simulink model "dspwavelet_frame2"  (R2016b)
settings: Solver=FixedStepDiscrete  StartTime=0.0  StopTime=1024  FixedStep=1e-5  RelTol=1e-3  EnableMultiTasking=on
undefined symbols (not defined in the file or in its folder): lod, ts
libraries: dspsrcs4 x3, dspmlti4 x2, dspmisc x1
settings Model: ExtModeTrigMode=oneshot  ExtModeArmWhenConnect=off  Creator=The MathWorks, Inc.  LastModifiedBy=admin
settings DataIOCC: SaveFormat=Array  SaveOutput=off  SaveTime=off  SignalLoggingName=sigsOut
settings OptimizationCC: BlockReduction=off  BooleanDataType=off  ExpressionDepthLimit=2147483647  InitFltsAndDblsToZero=on  EfficientMapNaN2IntZero=off  LifeSpan=inf
settings DebuggingCC: SaveWithParameterizedLinksMsg=none  UnderspecifiedInitializationDetection=Classic  MergeDetectMultiDrivingBlocksExec=none  SignalResolutionControl=TryResolveAllWithWarning  MultiTaskDSMMsg=warning  MultiTaskCondExecSysMsg=none  IntegerOverflowMsg=none  FcnCallInpInsideContextMsg=warning  StateNameClashWarn=warning  SFUnexpectedBacktrackingDiag=warning  SFNoUnconditionalDefaultTransitionDiag=warning  SFExecutionAtInitializationDiag=none  IntegerSaturationMsg=none
settings HardwareCC: ProdBitPerPointer=32  ProdBitPerSizeT=32  ProdBitPerPtrDiffT=32  ProdLargestAtomicFloat=None  ProdIntDivRoundTo=Undefined  ProdEndianess=Unspecified  ProdWordSize=32  ProdHWDeviceType=32-bit Generic  TargetUnknown=on
settings ModelReferenceCC: PropagateSignalLabelsOutOfModel=off
settings GRTTargetCC: TargetFcnLib=ansi_tfl_tmw.mat  TargetLangStandard=C89/C90 (ANSI)  GeneratePreprocessorConditionals=Disable all  CombineOutputUpdateFcns=off  GRTInterface=on
settings ConfigComp: CovMetricSettings=dw  CovHtmlReporting=on  CovSaveCumulativeToWorkspaceVar=on  CovSaveSingleToWorkspaceVar=on  CovExternalEMLEnable=off  CovSFcnEnable=off

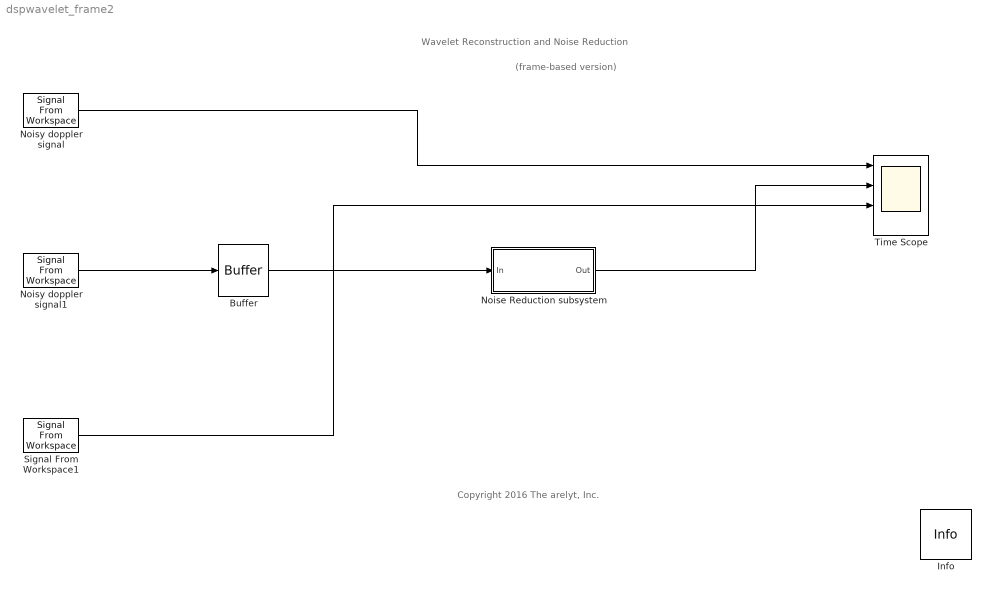
== system dspwavelet_frame2 ==
  note: Wavelet Reconstruction and Noise Reduction
  note: Copyright 2016 The arelyt, Inc.
  note: (frame-based version)
  Buffer : Buffer  TreatMby1Signals=One channel  OutputFrames=off
  Info : dspmisc/Info  SystemSampleTime=-1
  Noise Reduction subsystem : Subsystem  TreatAsAtomicUnit=on
  Noisy doppler signal : dspsrcs4/Signal From Workspace  X=signal  Ts=ts  nsamps=1  OutputAfterFinalValue=Holding final value  ignoreOrWarnInputAndFrameLengths=off  OutputFrames=off
  Noisy doppler signal1 : dspsrcs4/Signal From Workspace  X=signal  Ts=ts  nsamps=64  OutputAfterFinalValue=Holding final value  ignoreOrWarnInputAndFrameLengths=off  OutputFrames=off
  Signal From Workspace1 : dspsrcs4/Signal From Workspace  X=price  Ts=ts  nsamps=1  OutputAfterFinalValue=Holding final value  ignoreOrWarnInputAndFrameLengths=off  OutputFrames=off
  Time Scope : Scope  NumInputPorts=4
  wires:
  Noisy doppler signal/1 -> Time Scope/1
  Signal From Workspace1/1 -> Time Scope/3
  Noisy doppler signal1/1 -> Buffer/1
  Noise Reduction subsystem/1(Out) -> Time Scope/2
  Buffer/1 -> Noise Reduction subsystem/1(In)

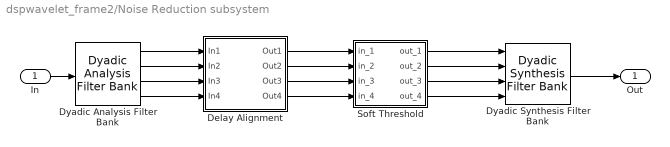
== system dspwavelet_frame2/Noise Reduction subsystem ==
  In : Inport
  Delay Alignment : Subsystem
  Dyadic Analysis Filter Bank : dspmlti4/Dyadic Analysis Filter Bank  Wname=User-defined  OrdRec_ordDec=[1 / 1]  Order=2  LPF=lod  HPF=hid  NumLevels=3  tree=Asymmetric  Output=Multiple ports  OutputFrames=off
  Dyadic Synthesis Filter Bank : dspmlti4/Dyadic Synthesis Filter Bank  Wname=User-defined  OrdRec_ordDec=[1 / 1]  Order=2  LPF=lor  HPF=hir  NumLevels=3  tree=Asymmetric  Input=Multiple ports  OutputFrames=off
  Soft Threshold : Subsystem  mask(Soft Threshold){st=[3 2 1 0]}
      mask prompts: st "Vector of thresholds for each level:"
      mask help: Apply a soft threshold (deadzone transfer function) to each signal in the decomposition. First threshold applies to top-most filter bank output.
      mask init:
      | x=([-1 1 NaN 0 0 NaN -1 -.5 .5 1]+1)/2*.7+.15;
      | y=([0 0 NaN -1 1 NaN -1 0 0 1]+1)/2*.7+.05;
      mask Help: Vector of thresholds for each decomposition level.
      mask Display:
      | text(.1,.9,'Dead Zone')
      | plot(x,y)
  Out : Outport
  wires:
  In/1 -> Dyadic Analysis Filter Bank/1
  Dyadic Synthesis Filter Bank/1 -> Out/1
  Dyadic Analysis Filter Bank/2 -> Delay Alignment/2(In2)
  Dyadic Analysis Filter Bank/1 -> Delay Alignment/1(In1)
  Delay Alignment/2(Out2) -> Soft Threshold/2(in_2)
  Delay Alignment/1(Out1) -> Soft Threshold/1(in_1)
  Soft Threshold/1(out_1) -> Dyadic Synthesis Filter Bank/1
  Soft Threshold/2(out_2) -> Dyadic Synthesis Filter Bank/2
  Dyadic Analysis Filter Bank/3 -> Delay Alignment/3(In3)
  Dyadic Analysis Filter Bank/4 -> Delay Alignment/4(In4)
  Delay Alignment/3(Out3) -> Soft Threshold/3(in_3)
  Delay Alignment/4(Out4) -> Soft Threshold/4(in_4)
  Soft Threshold/3(out_3) -> Dyadic Synthesis Filter Bank/3
  Soft Threshold/4(out_4) -> Dyadic Synthesis Filter Bank/4

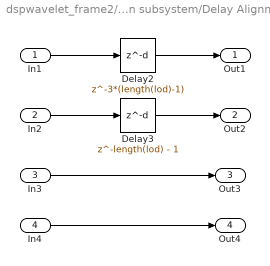
== system dspwavelet_frame2/Noise Reduction subsystem/Delay Alignment ==
  In1 : Inport
  In2 : Inport  Port=2
  In3 : Inport  Port=3
  In4 : Inport  Port=4
  Delay2 : Delay  DelayLength=3*(length(lod)-1)  InputProcessing=Columns as channels (frame based)
  Delay3 : Delay  DelayLength=length(lod) - 1  InputProcessing=Columns as channels (frame based)
  Out1 : Outport
  Out2 : Outport  Port=2
  Out3 : Outport  Port=3
  Out4 : Outport  Port=4
  wires:
  In3/1 -> Out3/1
  In4/1 -> Out4/1
  In2/1 -> Delay3/1
  Delay3/1 -> Out2/1
  In1/1 -> Delay2/1
  Delay2/1 -> Out1/1

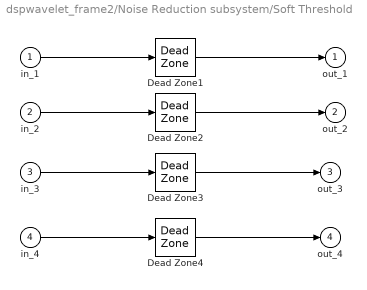
== system dspwavelet_frame2/Noise Reduction subsystem/Soft Threshold ==
  in_1 : Inport
  in_2 : Inport  Port=2
  in_3 : Inport  Port=3
  in_4 : Inport  Port=4
  Dead Zone1 : DeadZone  LowerValue=-st(1)  UpperValue=st(1)  ZeroCross=off  SaturateOnIntegerOverflow=on
  Dead Zone2 : DeadZone  LowerValue=-st(2)  UpperValue=st(2)  ZeroCross=off  SaturateOnIntegerOverflow=on
  Dead Zone3 : DeadZone  LowerValue=-st(3)  UpperValue=st(3)  ZeroCross=off  SaturateOnIntegerOverflow=on
  Dead Zone4 : DeadZone  LowerValue=-st(4)  UpperValue=st(4)  ZeroCross=off  SaturateOnIntegerOverflow=on
  out_1 : Outport
  out_2 : Outport  Port=2
  out_3 : Outport  Port=3
  out_4 : Outport  Port=4
  wires:
  in_1/1 -> Dead Zone1/1
  in_2/1 -> Dead Zone2/1
  in_3/1 -> Dead Zone3/1
  in_4/1 -> Dead Zone4/1
  Dead Zone1/1 -> out_1/1
  Dead Zone2/1 -> out_2/1
  Dead Zone3/1 -> out_3/1
  Dead Zone4/1 -> out_4/1
